simulink model "sss"  (R2015a)
settings: Solver=ode45  StartTime=0.0  StopTime=10.0  RelTol=1e-3
undefined symbols (not defined in the file or in its folder): fdesignblkfcn, gcbh
settings Model: Creator=dell  LastModifiedBy=dell

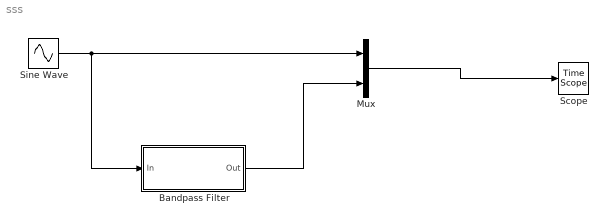
== system sss ==
  Bandpass Filter : Subsystem  DialogController=fdesignblkfcn  InitFcn=fdesignblkfcn(gcbh, {'InitFcn'});  mask(Bandpass Filter){}
      mask help: Design a bandpass filter
      settings: CopyFcn=fdesignblkfcn(gcbh, {'CopyFcn'});
      mask Help: helpview(mapfilelocation('dsp'), 'dspbandpassfilter');
      mask Display: disp('Bandpass');
  Mux : Mux  Inputs=2
  Scope : TimeScope
  Sine Wave : Sin  SampleTime=0
  wires:
  Sine Wave/1 -> Bandpass Filter/1(In), Mux/1
  Mux/1 -> Scope/1
  Bandpass Filter/1(Out) -> Mux/2

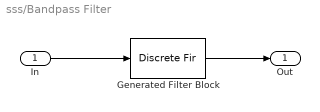
== system sss/Bandpass Filter ==
  In : Inport
  Generated Filter Block : DiscreteFir  Tag=BlockMethodSubSystem  Coefficients=[0.0025183893539179958 -0.0053669169258668331 0.0030675262786950021 0.0062122739003438922 -0.01349617201858744 0.0085789987278149619 0.0030372064102510438 -0.0045532941419756112 -0.0051763705962230566 0.0038539385318007418 0.020238137630203743 -0.039908869399416701 0.021578528882430989 0.018760147114490651 -0.02946454669394466 0.0043923408362241262 -0.0059973041405415976 0.068347251621229926 -0.11193379611063028 0.026502710816428271 0.15643409209427464 -0.25010470234972709 0.12281899806433721 0.12281899806433721 -0.25010470234972709 0.15643409209427464 0.026502710816428271 -0.11193379611063028 0.068347251621229926 -0.0059973041405415976 0.0043923408362241262 -0.02946454669394466 0.018760147114490651 0.021578528882430989 -0.039908869399416701 0.020238137630203743 0.0038539385318007418 -0.0051763705962230566 -0.0045532941419756112 0.0030372064102510438 0.0085789987278149619 -0.01349617201858744 0.0062122739003438922 0.0030675262786950021 -0.0053669169258668331 0.0025183893539179958]  InputProcessing=Columns as channels (frame based)
  Out : Outport
  wires:
  In/1 -> Generated Filter Block/1
  Generated Filter Block/1 -> Out/1
